simulink model "Relay_Blocks"  (Simulink 7.8)
settings: Solver=ode45  StartTime=0.0  StopTime=10.0  RelTol=1e-3
PreLoadFcn:
  | Ts = 1;
InitFcn:
  | Ts = 1;
undefined symbols (not defined in the file or in its folder): breakers_1ph_3ph, DiscIntNeverNeededParam, IEEE_Std_C37_112
libraries: simulink x12, powerlib_extras x8, lib_Timer_Counter x7, simulink_extras x3, dspsigops x1
settings Model: Creator=ma25949  LastModifiedBy=ma25949

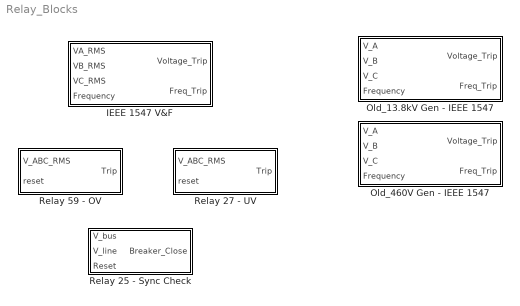
== system Relay_Blocks ==
  IEEE 1547 V&F : Subsystem  mask{V=13800, OF1=2, OF2=0.16, OV1=1, OV2=0.16, UF1=0.16, UF2=2, UV1=0.16, UV2=1, UV3=2}
      mask prompts: V "VoltageLL_RMS"; OF1 "OF1 (>60.5 Hz)"; OF2 "OF2 (>62 Hz)"; OV1 "OV1 (110% <V< 120% Vnom"; OV2 "OV2 (120% Vnom)"; UF1 "UF1 (<57 Hz)"; UF2 "UF2 (<59.5 Hz)"; UV1 "UV1 (<45% Vnom)"; UV2 "UV2 (45%<V<60% Vnom)"; UV3 "UV3 (60%<V<88% Vnom)"
      mask help:
      | This block implements interconnection system response according to IEEE Std. 1547-2014a.
      |
      | Fields to be filled are clearing times in seconds.
  Old_13.8kV Gen - IEEE 1547 : Subsystem  mask{OF1=2, OF2=0.16, OV1=1, OV2=0.16, UF1=0.16, UF2=2, UV1=0.16, UV2=1, UV3=2}
      mask prompts: OF1 "OF1 (>60.5 Hz)"; OF2 "OF2 (>62 Hz)"; OV1 "OV1 (110%<V<120% Vnom)"; OV2 "OV2 (>120% Vnom)"; UF1 "UF1 (<57 Hz)"; UF2 "UF2 (<59.5 Hz)"; UV1 "UV1 (<45% Vnom)"; UV2 "UV2 (45%<V<60% Vnom)"; UV3 "UV3 (60%<V<88% Vnom)"
      mask help:
      | This block implements interconnection system response according to IEEE Std. 1547-2014a.
      |
      | Fields to be filled are clearing times in seconds.
  Old_460V Gen - IEEE 1547 : Subsystem  mask{OF1=2, OF2=0.16, OV1=1, OV2=0.16, UF1=0.16, UF2=2, UV1=0.16, UV2=1, UV3=2}
      mask prompts: OF1 "OF1 (>60.5 Hz)"; OF2 "OF2 (>62 Hz)"; OV1 "OV1 (110%<V<120% Vnom)"; OV2 "OV2 (>120% Vnom)"; UF1 "UF1 (<57 Hz)"; UF2 "UF2 (<59.5 Hz)"; UV1 "UV1 (<45% Vnom)"; UV2 "UV2 (45%<V<60% Vnom)"; UV3 "UV3 (60%<V<88% Vnom)"
      mask help:
      | This block implements interconnection system response according to IEEE Std. 1547-2014a.
      |
      | Fields to be filled are clearing times in seconds.
  Relay 25 - Sync Check : Subsystem  mask{Cycles=2, V=13800}
      mask prompts: Cycles "# of cycles to check for sync"; V "VRMS_NominalV"
  Relay 27 - UV : Subsystem  mask{V=13800}
      mask prompts: V "Vnom"
      mask help: TOV Pickup is set to +15% of Vnominal.
  Relay 59 - OV : Subsystem  mask{V=13800}
      mask prompts: V "Vnom"
      mask help: TOV Pickup is set to +15% of Vnominal.

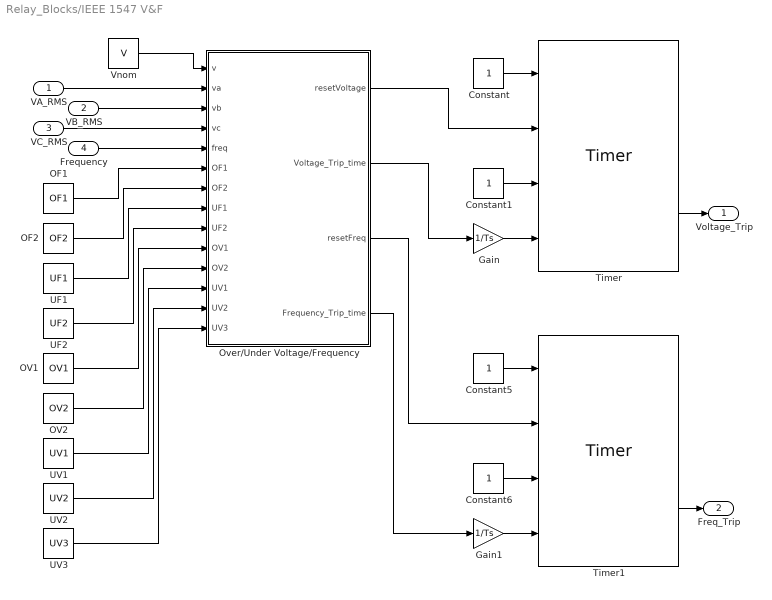
== system Relay_Blocks/IEEE 1547 V&F ==
  VA_RMS : Inport
  VB_RMS : Inport  Port=2
  VC_RMS : Inport  Port=3
  Frequency : Inport  Port=4
  Constant{,1,5..6} (4 alike) : Constant
  Gain : Gain  Gain=1/Ts
  Gain1 : Gain  Gain=1/Ts
  OF1 : Constant  Value=OF1
  OF2 : Constant  Value=OF2
  OV1 : Constant  Value=OV1
  OV2 : Constant  Value=OV2
  Over/Under Voltage/Frequency : MATLAB Function  TreatAsAtomicUnit=on
  Timer : lib_Timer_Counter/Timer
  Timer1 : lib_Timer_Counter/Timer
  UF1 : Constant  Value=UF1
  UF2 : Constant  Value=UF2
  UV1 : Constant  Value=UV1
  UV2 : Constant  Value=UV2
  UV3 : Constant  Value=UV3
  Vnom : Constant  Value=V
  Voltage_Trip : Outport
  Freq_Trip : Outport  Port=2
  wires:
  Constant/1 -> Timer/1
  Constant1/1 -> Timer/3
  Constant5/1 -> Timer1/1
  Constant6/1 -> Timer1/3
  Timer/2 -> Voltage_Trip/1
  Timer1/2 -> Freq_Trip/1
  VA_RMS/1 -> Over/Under Voltage/Frequency/2(va)
  Vnom/1 -> Over/Under Voltage/Frequency/1(v)
  VB_RMS/1 -> Over/Under Voltage/Frequency/3(vb)
  VC_RMS/1 -> Over/Under Voltage/Frequency/4(vc)
  Frequency/1 -> Over/Under Voltage/Frequency/5(freq)
  Over/Under Voltage/Frequency/1(resetVoltage) -> Timer/2
  Over/Under Voltage/Frequency/3(resetFreq) -> Timer1/2
  Gain1/1 -> Timer1/4
  Gain/1 -> Timer/4
  Over/Under Voltage/Frequency/2(Voltage_Trip_time) -> Gain/1
  Over/Under Voltage/Frequency/4(Frequency_Trip_time) -> Gain1/1
  OF1/1 -> Over/Under Voltage/Frequency/6(OF1)
  OF2/1 -> Over/Under Voltage/Frequency/7(OF2)
  UF1/1 -> Over/Under Voltage/Frequency/8(UF1)
  UF2/1 -> Over/Under Voltage/Frequency/9(UF2)
  OV1/1 -> Over/Under Voltage/Frequency/10(OV1)
  OV2/1 -> Over/Under Voltage/Frequency/11(OV2)
  UV1/1 -> Over/Under Voltage/Frequency/12(UV1)
  UV2/1 -> Over/Under Voltage/Frequency/13(UV2)
  UV3/1 -> Over/Under Voltage/Frequency/14(UV3)

== system Relay_Blocks/Old_13.8kV Gen - IEEE 1547 ==
  V_A : Inport
  V_B : Inport  Port=2
  V_C : Inport  Port=3
  Frequency : Inport  Port=4
  " Min_ClearingTime" : MinMax  Inputs=3
  Constant{,1,5..6} (4 alike) : Constant
  Frequency1 : Subsystem
  Logical Operator : Logic  Inputs=3  AllPortsSameDT=off  OutDataTypeStr=boolean
  PhaseA : Subsystem
  PhaseB : Subsystem
  PhaseC : Subsystem
  Timer : lib_Timer_Counter/Timer
  Timer1 : lib_Timer_Counter/Timer
  Voltage_Trip : Outport
  Freq_Trip : Outport  Port=2
  wires:
  Constant/1 -> Timer/1
  Constant1/1 -> Timer/3
  Constant5/1 -> Timer1/1
  Constant6/1 -> Timer1/3
  Frequency/1 -> Frequency1/1(Freq)
  Timer/2 -> Voltage_Trip/1
  Timer1/2 -> Freq_Trip/1
  V_A/1 -> PhaseA/1(V)
  V_B/1 -> PhaseB/1(V)
  V_C/1 -> PhaseC/1(V)
  PhaseA/2(Target Time) -> " Min_ClearingTime"/1
  " Min_ClearingTime"/1 -> Timer/4
  PhaseA/1(Reset) -> Logical Operator/1
  Logical Operator/1 -> Timer/2
  PhaseB/1(Reset) -> Logical Operator/2
  PhaseC/1(Reset) -> Logical Operator/3
  PhaseB/2(Target Time) -> " Min_ClearingTime"/2
  PhaseC/2(Target Time) -> " Min_ClearingTime"/3
  Frequency1/1(Reset) -> Timer1/2
  Frequency1/2(Target Time) -> Timer1/4

== system Relay_Blocks/Old_460V Gen - IEEE 1547 ==
  V_A : Inport
  V_B : Inport  Port=2
  V_C : Inport  Port=3
  Frequency : Inport  Port=4
  " Min_ClearingTime" : MinMax  Inputs=3
  Constant{,1,5..6} (4 alike) : Constant
  Frequency1 : Subsystem
  Logical Operator : Logic  Inputs=3  AllPortsSameDT=off  OutDataTypeStr=boolean
  PhaseA : Subsystem
  PhaseB : Subsystem
  PhaseC : Subsystem
  Timer : lib_Timer_Counter/Timer
  Timer1 : lib_Timer_Counter/Timer
  Voltage_Trip : Outport
  Freq_Trip : Outport  Port=2
  wires:
  Constant/1 -> Timer/1
  Constant1/1 -> Timer/3
  Constant5/1 -> Timer1/1
  Constant6/1 -> Timer1/3
  Frequency/1 -> Frequency1/1(Freq)
  Timer/2 -> Voltage_Trip/1
  Timer1/2 -> Freq_Trip/1
  V_A/1 -> PhaseA/1(V)
  V_B/1 -> PhaseB/1(V)
  V_C/1 -> PhaseC/1(V)
  PhaseA/2(Target Time) -> " Min_ClearingTime"/1
  " Min_ClearingTime"/1 -> Timer/4
  PhaseA/1(Reset) -> Logical Operator/1
  Logical Operator/1 -> Timer/2
  PhaseB/1(Reset) -> Logical Operator/2
  PhaseC/1(Reset) -> Logical Operator/3
  PhaseB/2(Target Time) -> " Min_ClearingTime"/2
  PhaseC/2(Target Time) -> " Min_ClearingTime"/3
  Frequency1/1(Reset) -> Timer1/2
  Frequency1/2(Target Time) -> Timer1/4

== system Relay_Blocks/Relay 25 - Sync Check ==
  V_bus : Inport
  V_line : Inport  Port=2
  Reset : Inport  Port=3
  Compare To Constant3 : simulink/Logic and Bit Operations/Compare To Constant  relop===  const=0  OutDataTypeStr=uint8
  Constant : Constant
  Freq_Comparator : Subsystem
  Gain : Gain  Gain=0.16667/Ts
  Logical Operator : Logic  Inputs=3  AllPortsSameDT=off  OutDataTypeStr=boolean
  Logical Operator1 : Logic  Operator=OR  AllPortsSameDT=off  OutDataTypeStr=boolean
  Phase_Comparator : Subsystem
  RMS Calculator1 : Subsystem
  RMS Calculator2 : Subsystem
  Subsystem : Subsystem
  Target_time : Constant  Value=Cycles
  Timer : lib_Timer_Counter/Timer
  Voltage_Comparator : Subsystem
  Breaker_Close : Outport
  wires:
  Logical Operator/1 -> Compare To Constant3/1, Timer/1
  Constant/1 -> Timer/3
  Phase_Comparator/2(Locked) -> Logical Operator/3
  Freq_Comparator/2(Locked) -> Logical Operator/2
  Voltage_Comparator/3(Locked) -> Logical Operator/1
  RMS Calculator1/1(VRMSLL) -> Voltage_Comparator/2(V_line)
  Subsystem/4(wt_line) -> Phase_Comparator/2(wt_line)
  Subsystem/3(wt_bus) -> Phase_Comparator/1(wt_bus)
  Subsystem/2(f_line) -> Freq_Comparator/2(f_line)
  Subsystem/1(f_bus) -> Freq_Comparator/1(f_bus)
  V_line/1 -> Subsystem/2(V_line), RMS Calculator1/1(Vpeak)
  V_bus/1 -> Subsystem/1(V_bus), RMS Calculator2/1(Vpeak)
  Timer/2 -> Breaker_Close/1
  RMS Calculator2/1(VRMSLL) -> Voltage_Comparator/1(V_bus)
  ? -> [Mode]
  Target_time/1 -> Gain/1
  Gain/1 -> Timer/4
  Reset/1 -> Logical Operator1/1
  Logical Operator1/1 -> Timer/2
  Compare To Constant3/1 -> Logical Operator1/2

== system Relay_Blocks/Relay 27 - UV ==
  V_ABC_RMS : Inport
  reset : Inport  Port=2
  Data Type Conversion1 : DataTypeConversion
  Data Type Conversion3 : DataTypeConversion
  Demux : Demux  Outputs=3
  Demux1 : Demux  Outputs=3
  Discrete-Time Integrator1 : DiscreteIntegrator  IntegratorMethod=Integration: Trapezoidal  ExternalReset=falling  InitialConditionMode=State only (most efficient)  SampleTime=-1  ICPrevOutput=DiscIntNeverNeededParam  ICPrevScaledInput=DiscIntNeverNeededParam
  Gain : Gain  Gain=0.85
  Logical Operator1 : Logic  Operator=OR  Inputs=3  AllPortsSameDT=off  OutDataTypeStr=boolean
  Relational Operator : RelationalOperator  Operator=<  OutDataTypeStr=boolean
  Relational Operator1 : RelationalOperator  Operator=>  OutDataTypeStr=boolean
  S-R Flip-Flop : simulink_extras/Flip Flops/S-R Flip-Flop  initial_condition=0
  Terminator : Terminator
  UV Relay : Subsystem  AncestorBlock=breakers_1ph_3ph/IEEE_Std_C37_112
  Vnom : Constant  Value=V
  Trip : Outport
  wires:
  Data Type Conversion1/1 -> Discrete-Time Integrator1/1
  UV Relay/1(T_trip) -> Relational Operator/1  "t_trip"
  Demux/1 -> UV Relay/2(Va)
  Demux/2 -> UV Relay/3(Vb)
  Demux/3 -> UV Relay/4(Vc)
  V_ABC_RMS/1 -> Demux/1, Relational Operator1/2
  S-R Flip-Flop/1 -> Trip/1
  S-R Flip-Flop/2 -> Terminator/1
  reset/1 -> Data Type Conversion3/1
  Data Type Conversion3/1 -> S-R Flip-Flop/2
  Relational Operator1/1 -> Data Type Conversion1/1, Discrete-Time Integrator1/2
  Discrete-Time Integrator1/1 -> Relational Operator/2
  Vnom/1 -> Gain/1
  Gain/1 -> UV Relay/1(TOV_pickup), Relational Operator1/1
  Relational Operator/1 -> Demux1/1
  Demux1/1 -> Logical Operator1/1
  Demux1/2 -> Logical Operator1/2
  Demux1/3 -> Logical Operator1/3
  Logical Operator1/1 -> S-R Flip-Flop/1

== system Relay_Blocks/Relay 59 - OV ==
  V_ABC_RMS : Inport
  reset : Inport  Port=2
  Data Type Conversion1 : DataTypeConversion
  Data Type Conversion3 : DataTypeConversion
  Demux : Demux  Outputs=3
  Demux1 : Demux  Outputs=3
  Discrete-Time Integrator1 : DiscreteIntegrator  IntegratorMethod=Integration: Trapezoidal  ExternalReset=falling  InitialConditionMode=State only (most efficient)  SampleTime=-1  ICPrevOutput=DiscIntNeverNeededParam  ICPrevScaledInput=DiscIntNeverNeededParam
  Gain : Gain  Gain=1.15
  Logical Operator1 : Logic  Operator=OR  Inputs=3  AllPortsSameDT=off  OutDataTypeStr=boolean
  OV Relay : Subsystem  AncestorBlock=breakers_1ph_3ph/IEEE_Std_C37_112
  Relational Operator : RelationalOperator  Operator=<  OutDataTypeStr=boolean
  Relational Operator1 : RelationalOperator  Operator=<  OutDataTypeStr=boolean
  S-R Flip-Flop : simulink_extras/Flip Flops/S-R Flip-Flop  initial_condition=0
  Terminator : Terminator
  Vnom : Constant  Value=V
  Trip : Outport
  wires:
  Data Type Conversion1/1 -> Discrete-Time Integrator1/1
  OV Relay/1(T_trip) -> Relational Operator/1  "t_trip"
  Demux/1 -> OV Relay/2(Va)
  Demux/2 -> OV Relay/3(Vb)
  Demux/3 -> OV Relay/4(Vc)
  V_ABC_RMS/1 -> Demux/1, Relational Operator1/2
  S-R Flip-Flop/1 -> Trip/1
  S-R Flip-Flop/2 -> Terminator/1
  reset/1 -> Data Type Conversion3/1
  Data Type Conversion3/1 -> S-R Flip-Flop/2
  Relational Operator1/1 -> Data Type Conversion1/1, Discrete-Time Integrator1/2
  Discrete-Time Integrator1/1 -> Relational Operator/2
  Vnom/1 -> Gain/1
  Gain/1 -> OV Relay/1(TOV_pickup), Relational Operator1/1
  Relational Operator/1 -> Demux1/1
  Demux1/1 -> Logical Operator1/1
  Demux1/2 -> Logical Operator1/2
  Demux1/3 -> Logical Operator1/3
  Logical Operator1/1 -> S-R Flip-Flop/1

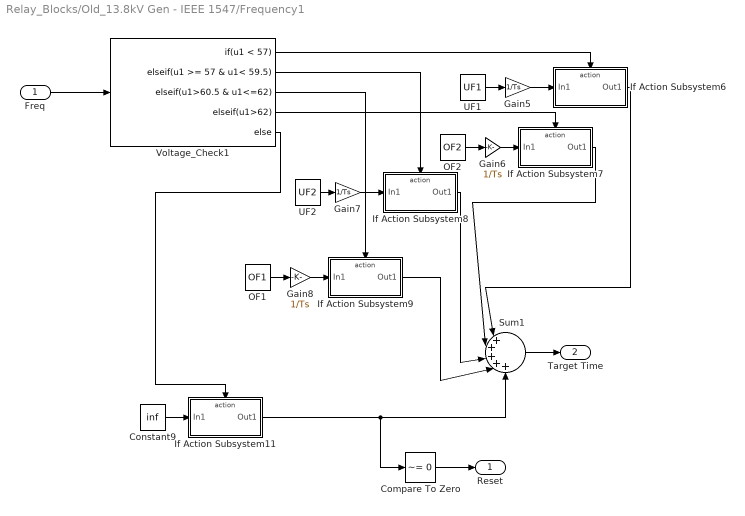
== system Relay_Blocks/Old_13.8kV Gen - IEEE 1547/Frequency1 ==
  Freq : Inport
  Compare To Zero : simulink/Logic and Bit Operations/Compare To Zero  relop=~=  OutDataTypeStr=uint8
  Constant9 : Constant  Value=inf
  Gain{5..8} (4 alike) : Gain  Gain=1/Ts
  If Action Subsystem11 : Subsystem  TreatAsAtomicUnit=on
  If Action Subsystem6 : Subsystem  TreatAsAtomicUnit=on
  If Action Subsystem7 : Subsystem  TreatAsAtomicUnit=on
  If Action Subsystem8 : Subsystem  TreatAsAtomicUnit=on
  If Action Subsystem9 : Subsystem  TreatAsAtomicUnit=on
  OF1 : Constant  Value=OF1
  OF2 : Constant  Value=OF2
  Sum1 : Sum  Inputs=|+++++
  UF1 : Constant  Value=UF1
  UF2 : Constant  Value=UF2
  Voltage_Check1 : If  IfExpression=u1 < 57  ElseIfExpressions="u1 >= 57 & u1< 59.5,  u1>60.5 & u1<=62, u1>62"
  Reset : Outport
  Target Time : Outport  Port=2
  wires:
  Freq/1 -> Voltage_Check1/1
  Voltage_Check1/1 -> If Action Subsystem6/Action
  UF1/1 -> Gain5/1
  Voltage_Check1/4 -> If Action Subsystem7/Action
  Voltage_Check1/2 -> If Action Subsystem8/Action
  Voltage_Check1/3 -> If Action Subsystem9/Action
  UF2/1 -> Gain7/1
  Voltage_Check1/5 -> If Action Subsystem11/Action
  Constant9/1 -> If Action Subsystem11/1(In1)
  If Action Subsystem6/1(Out1) -> Sum1/1
  If Action Subsystem7/1(Out1) -> Sum1/2
  If Action Subsystem8/1(Out1) -> Sum1/3
  If Action Subsystem9/1(Out1) -> Sum1/4
  If Action Subsystem11/1(Out1) -> Sum1/5, Compare To Zero/1
  OF1/1 -> Gain8/1
  OF2/1 -> Gain6/1
  Gain5/1 -> If Action Subsystem6/1(In1)
  Gain6/1 -> If Action Subsystem7/1(In1)
  Gain7/1 -> If Action Subsystem8/1(In1)
  Gain8/1 -> If Action Subsystem9/1(In1)
  Sum1/1 -> Target Time/1
  Compare To Zero/1 -> Reset/1

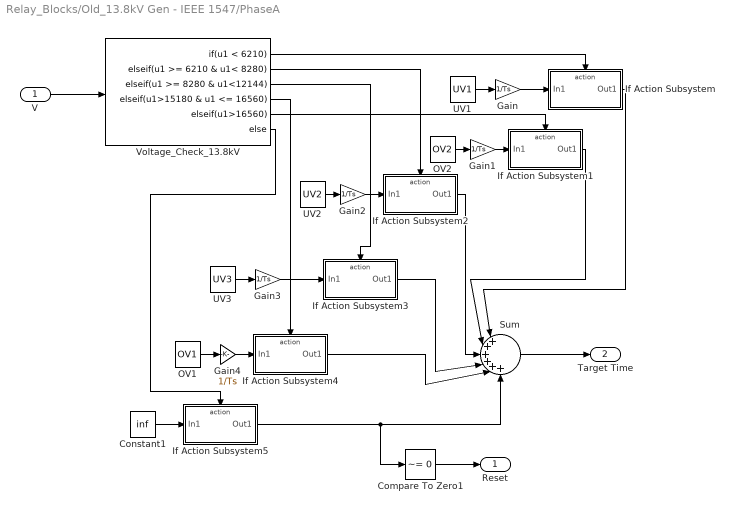
== system Relay_Blocks/Old_13.8kV Gen - IEEE 1547/PhaseA ==
  V : Inport
  Compare To Zero1 : simulink/Logic and Bit Operations/Compare To Zero  relop=~=  OutDataTypeStr=uint8
  Constant1 : Constant  Value=inf
  Gain{,1..4} (5 alike) : Gain  Gain=1/Ts
  If Action Subsystem : Subsystem  TreatAsAtomicUnit=on
  If Action Subsystem1 : Subsystem  TreatAsAtomicUnit=on
  If Action Subsystem2 : Subsystem  TreatAsAtomicUnit=on
  If Action Subsystem3 : Subsystem  TreatAsAtomicUnit=on
  If Action Subsystem4 : Subsystem  TreatAsAtomicUnit=on
  If Action Subsystem5 : Subsystem  TreatAsAtomicUnit=on
  OV1 : Constant  Value=OV1
  OV2 : Constant  Value=OV2
  Sum : Sum  Inputs=|++++++
  UV1 : Constant  Value=UV1
  UV2 : Constant  Value=UV2
  UV3 : Constant  Value=UV3
  Voltage_Check_13.8kV : If  IfExpression=u1 < 6210  ElseIfExpressions="u1 >= 6210 & u1< 8280,  u1 >= 8280 & u1<12144, u1>15180 & u1 <= 16560, u1>16560"
  Reset : Outport
  Target Time : Outport  Port=2
  wires:
  Voltage_Check_13.8kV/1 -> If Action Subsystem/Action
  Voltage_Check_13.8kV/5 -> If Action Subsystem1/Action
  Voltage_Check_13.8kV/2 -> If Action Subsystem2/Action
  Voltage_Check_13.8kV/3 -> If Action Subsystem3/Action
  Voltage_Check_13.8kV/4 -> If Action Subsystem4/Action
  UV3/1 -> Gain3/1
  Voltage_Check_13.8kV/6 -> If Action Subsystem5/Action
  Constant1/1 -> If Action Subsystem5/1(In1)
  If Action Subsystem/1(Out1) -> Sum/1
  If Action Subsystem1/1(Out1) -> Sum/2
  If Action Subsystem2/1(Out1) -> Sum/3
  If Action Subsystem3/1(Out1) -> Sum/4
  If Action Subsystem4/1(Out1) -> Sum/5
  If Action Subsystem5/1(Out1) -> Sum/6, Compare To Zero1/1
  OV1/1 -> Gain4/1
  UV1/1 -> Gain/1
  Gain/1 -> If Action Subsystem/1(In1)
  OV2/1 -> Gain1/1
  Gain1/1 -> If Action Subsystem1/1(In1)
  UV2/1 -> Gain2/1
  Gain2/1 -> If Action Subsystem2/1(In1)
  Gain3/1 -> If Action Subsystem3/1(In1)
  Gain4/1 -> If Action Subsystem4/1(In1)
  V/1 -> Voltage_Check_13.8kV/1
  Compare To Zero1/1 -> Reset/1
  Sum/1 -> Target Time/1

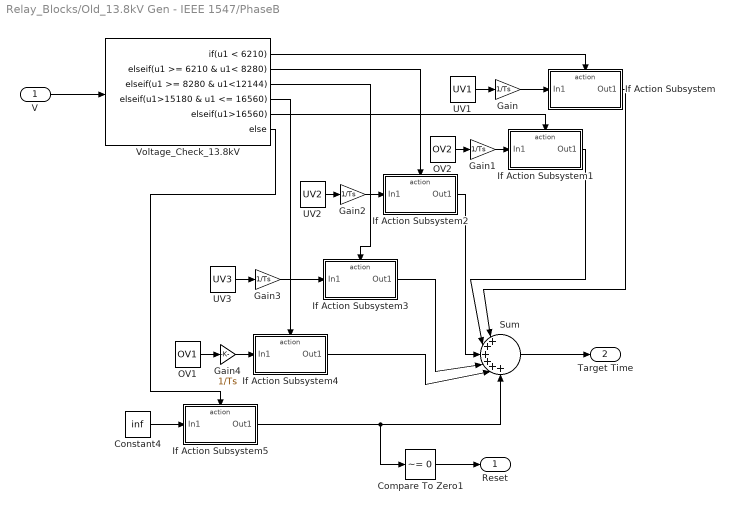
== system Relay_Blocks/Old_13.8kV Gen - IEEE 1547/PhaseB ==
  V : Inport
  Compare To Zero1 : simulink/Logic and Bit Operations/Compare To Zero  relop=~=  OutDataTypeStr=uint8
  Constant4 : Constant  Value=inf
  Gain{,1..4} (5 alike) : Gain  Gain=1/Ts
  If Action Subsystem : Subsystem  TreatAsAtomicUnit=on
  If Action Subsystem1 : Subsystem  TreatAsAtomicUnit=on
  If Action Subsystem2 : Subsystem  TreatAsAtomicUnit=on
  If Action Subsystem3 : Subsystem  TreatAsAtomicUnit=on
  If Action Subsystem4 : Subsystem  TreatAsAtomicUnit=on
  If Action Subsystem5 : Subsystem  TreatAsAtomicUnit=on
  OV1 : Constant  Value=OV1
  OV2 : Constant  Value=OV2
  Sum : Sum  Inputs=|++++++
  UV1 : Constant  Value=UV1
  UV2 : Constant  Value=UV2
  UV3 : Constant  Value=UV3
  Voltage_Check_13.8kV : If  IfExpression=u1 < 6210  ElseIfExpressions="u1 >= 6210 & u1< 8280,  u1 >= 8280 & u1<12144, u1>15180 & u1 <= 16560, u1>16560"
  Reset : Outport
  Target Time : Outport  Port=2
  wires:
  Voltage_Check_13.8kV/1 -> If Action Subsystem/Action
  Voltage_Check_13.8kV/5 -> If Action Subsystem1/Action
  Voltage_Check_13.8kV/2 -> If Action Subsystem2/Action
  Voltage_Check_13.8kV/3 -> If Action Subsystem3/Action
  Voltage_Check_13.8kV/4 -> If Action Subsystem4/Action
  UV3/1 -> Gain3/1
  Voltage_Check_13.8kV/6 -> If Action Subsystem5/Action
  Constant4/1 -> If Action Subsystem5/1(In1)
  If Action Subsystem/1(Out1) -> Sum/1
  If Action Subsystem1/1(Out1) -> Sum/2
  If Action Subsystem2/1(Out1) -> Sum/3
  If Action Subsystem4/1(Out1) -> Sum/5
  If Action Subsystem5/1(Out1) -> Sum/6, Compare To Zero1/1
  OV1/1 -> Gain4/1
  UV1/1 -> Gain/1
  Gain/1 -> If Action Subsystem/1(In1)
  OV2/1 -> Gain1/1
  Gain1/1 -> If Action Subsystem1/1(In1)
  UV2/1 -> Gain2/1
  Gain2/1 -> If Action Subsystem2/1(In1)
  Gain3/1 -> If Action Subsystem3/1(In1)
  Gain4/1 -> If Action Subsystem4/1(In1)
  V/1 -> Voltage_Check_13.8kV/1
  Compare To Zero1/1 -> Reset/1
  Sum/1 -> Target Time/1
  If Action Subsystem3/1(Out1) -> Sum/4

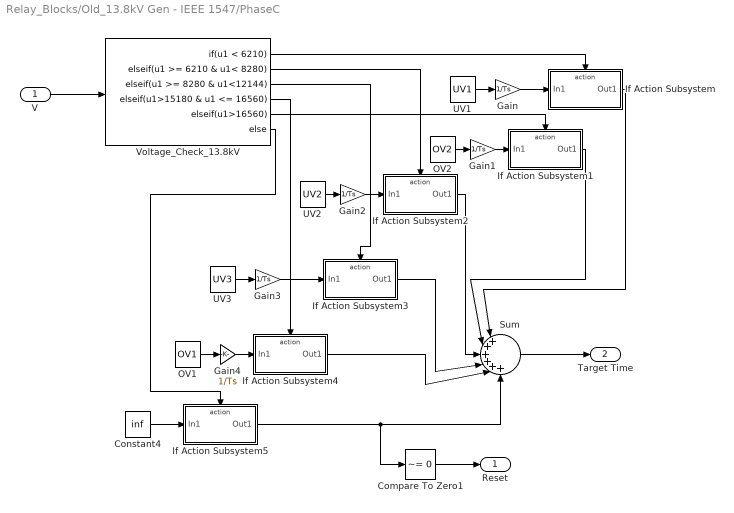
== system Relay_Blocks/Old_13.8kV Gen - IEEE 1547/PhaseC ==
  V : Inport
  Compare To Zero1 : simulink/Logic and Bit Operations/Compare To Zero  relop=~=  OutDataTypeStr=uint8
  Constant4 : Constant  Value=inf
  Gain{,1..4} (5 alike) : Gain  Gain=1/Ts
  If Action Subsystem : Subsystem  TreatAsAtomicUnit=on
  If Action Subsystem1 : Subsystem  TreatAsAtomicUnit=on
  If Action Subsystem2 : Subsystem  TreatAsAtomicUnit=on
  If Action Subsystem3 : Subsystem  TreatAsAtomicUnit=on
  If Action Subsystem4 : Subsystem  TreatAsAtomicUnit=on
  If Action Subsystem5 : Subsystem  TreatAsAtomicUnit=on
  OV1 : Constant  Value=OV1
  OV2 : Constant  Value=OV2
  Sum : Sum  Inputs=|++++++
  UV1 : Constant  Value=UV1
  UV2 : Constant  Value=UV2
  UV3 : Constant  Value=UV3
  Voltage_Check_13.8kV : If  IfExpression=u1 < 6210  ElseIfExpressions="u1 >= 6210 & u1< 8280,  u1 >= 8280 & u1<12144, u1>15180 & u1 <= 16560, u1>16560"
  Reset : Outport
  Target Time : Outport  Port=2
  wires:
  Voltage_Check_13.8kV/1 -> If Action Subsystem/Action
  Voltage_Check_13.8kV/5 -> If Action Subsystem1/Action
  Voltage_Check_13.8kV/2 -> If Action Subsystem2/Action
  Voltage_Check_13.8kV/3 -> If Action Subsystem3/Action
  Voltage_Check_13.8kV/4 -> If Action Subsystem4/Action
  UV3/1 -> Gain3/1
  Voltage_Check_13.8kV/6 -> If Action Subsystem5/Action
  Constant4/1 -> If Action Subsystem5/1(In1)
  If Action Subsystem/1(Out1) -> Sum/1
  If Action Subsystem1/1(Out1) -> Sum/2
  If Action Subsystem2/1(Out1) -> Sum/3
  If Action Subsystem3/1(Out1) -> Sum/4
  If Action Subsystem4/1(Out1) -> Sum/5
  If Action Subsystem5/1(Out1) -> Sum/6, Compare To Zero1/1
  OV1/1 -> Gain4/1
  UV1/1 -> Gain/1
  Gain/1 -> If Action Subsystem/1(In1)
  OV2/1 -> Gain1/1
  Gain1/1 -> If Action Subsystem1/1(In1)
  UV2/1 -> Gain2/1
  Gain2/1 -> If Action Subsystem2/1(In1)
  Gain3/1 -> If Action Subsystem3/1(In1)
  Gain4/1 -> If Action Subsystem4/1(In1)
  V/1 -> Voltage_Check_13.8kV/1
  Compare To Zero1/1 -> Reset/1
  Sum/1 -> Target Time/1

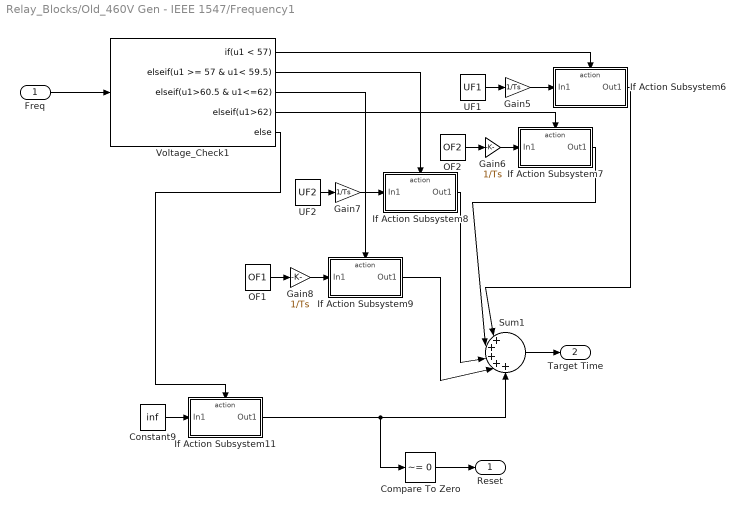
== system Relay_Blocks/Old_460V Gen - IEEE 1547/Frequency1 ==
  Freq : Inport
  Compare To Zero : simulink/Logic and Bit Operations/Compare To Zero  relop=~=  OutDataTypeStr=uint8
  Constant9 : Constant  Value=inf
  Gain{5..8} (4 alike) : Gain  Gain=1/Ts
  If Action Subsystem11 : Subsystem  TreatAsAtomicUnit=on
  If Action Subsystem6 : Subsystem  TreatAsAtomicUnit=on
  If Action Subsystem7 : Subsystem  TreatAsAtomicUnit=on
  If Action Subsystem8 : Subsystem  TreatAsAtomicUnit=on
  If Action Subsystem9 : Subsystem  TreatAsAtomicUnit=on
  OF1 : Constant  Value=OF1
  OF2 : Constant  Value=OF2
  Sum1 : Sum  Inputs=|+++++
  UF1 : Constant  Value=UF1
  UF2 : Constant  Value=UF2
  Voltage_Check1 : If  IfExpression=u1 < 57  ElseIfExpressions="u1 >= 57 & u1< 59.5,  u1>60.5 & u1<=62, u1>62"
  Reset : Outport
  Target Time : Outport  Port=2
  wires:
  Freq/1 -> Voltage_Check1/1
  Voltage_Check1/1 -> If Action Subsystem6/Action
  UF1/1 -> Gain5/1
  Voltage_Check1/4 -> If Action Subsystem7/Action
  Voltage_Check1/2 -> If Action Subsystem8/Action
  Voltage_Check1/3 -> If Action Subsystem9/Action
  UF2/1 -> Gain7/1
  Voltage_Check1/5 -> If Action Subsystem11/Action
  Constant9/1 -> If Action Subsystem11/1(In1)
  If Action Subsystem6/1(Out1) -> Sum1/1
  If Action Subsystem7/1(Out1) -> Sum1/2
  If Action Subsystem8/1(Out1) -> Sum1/3
  If Action Subsystem9/1(Out1) -> Sum1/4
  If Action Subsystem11/1(Out1) -> Sum1/5, Compare To Zero/1
  OF1/1 -> Gain8/1
  OF2/1 -> Gain6/1
  Gain5/1 -> If Action Subsystem6/1(In1)
  Gain6/1 -> If Action Subsystem7/1(In1)
  Gain7/1 -> If Action Subsystem8/1(In1)
  Gain8/1 -> If Action Subsystem9/1(In1)
  Sum1/1 -> Target Time/1
  Compare To Zero/1 -> Reset/1

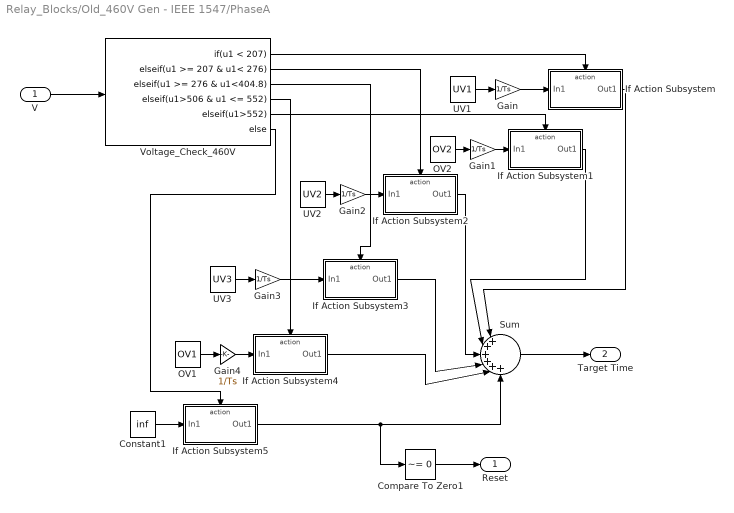
== system Relay_Blocks/Old_460V Gen - IEEE 1547/PhaseA ==
  V : Inport
  Compare To Zero1 : simulink/Logic and Bit Operations/Compare To Zero  relop=~=  OutDataTypeStr=uint8
  Constant1 : Constant  Value=inf
  Gain{,1..4} (5 alike) : Gain  Gain=1/Ts
  If Action Subsystem : Subsystem  TreatAsAtomicUnit=on
  If Action Subsystem1 : Subsystem  TreatAsAtomicUnit=on
  If Action Subsystem2 : Subsystem  TreatAsAtomicUnit=on
  If Action Subsystem3 : Subsystem  TreatAsAtomicUnit=on
  If Action Subsystem4 : Subsystem  TreatAsAtomicUnit=on
  If Action Subsystem5 : Subsystem  TreatAsAtomicUnit=on
  OV1 : Constant  Value=OV1
  OV2 : Constant  Value=OV2
  Sum : Sum  Inputs=|++++++
  UV1 : Constant  Value=UV1
  UV2 : Constant  Value=UV2
  UV3 : Constant  Value=UV3
  Voltage_Check_460V : If  IfExpression=u1 < 207  ElseIfExpressions="u1 >= 207 & u1< 276,  u1 >= 276 & u1<404.8, u1>506 & u1 <= 552, u1>552"
  Reset : Outport
  Target Time : Outport  Port=2
  wires:
  Voltage_Check_460V/1 -> If Action Subsystem/Action
  Voltage_Check_460V/5 -> If Action Subsystem1/Action
  Voltage_Check_460V/2 -> If Action Subsystem2/Action
  Voltage_Check_460V/3 -> If Action Subsystem3/Action
  Voltage_Check_460V/4 -> If Action Subsystem4/Action
  UV3/1 -> Gain3/1
  Voltage_Check_460V/6 -> If Action Subsystem5/Action
  Constant1/1 -> If Action Subsystem5/1(In1)
  If Action Subsystem/1(Out1) -> Sum/1
  If Action Subsystem1/1(Out1) -> Sum/2
  If Action Subsystem2/1(Out1) -> Sum/3
  If Action Subsystem3/1(Out1) -> Sum/4
  If Action Subsystem4/1(Out1) -> Sum/5
  If Action Subsystem5/1(Out1) -> Sum/6, Compare To Zero1/1
  OV1/1 -> Gain4/1
  UV1/1 -> Gain/1
  Gain/1 -> If Action Subsystem/1(In1)
  OV2/1 -> Gain1/1
  Gain1/1 -> If Action Subsystem1/1(In1)
  UV2/1 -> Gain2/1
  Gain2/1 -> If Action Subsystem2/1(In1)
  Gain3/1 -> If Action Subsystem3/1(In1)
  Gain4/1 -> If Action Subsystem4/1(In1)
  V/1 -> Voltage_Check_460V/1
  Compare To Zero1/1 -> Reset/1
  Sum/1 -> Target Time/1

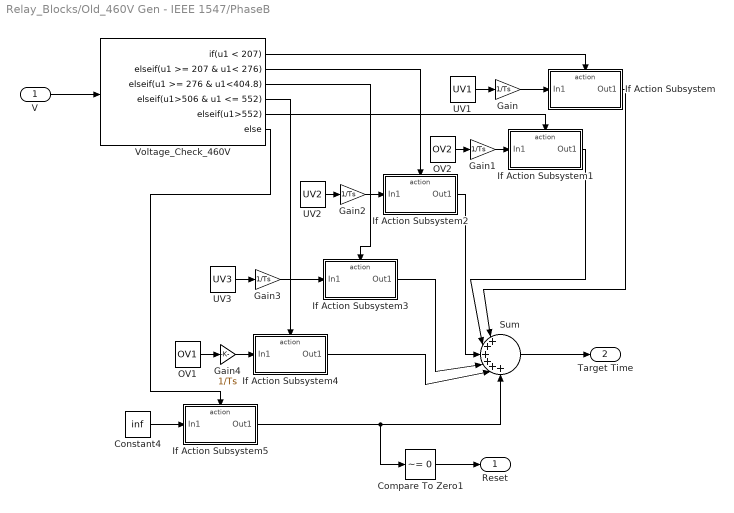
== system Relay_Blocks/Old_460V Gen - IEEE 1547/PhaseB ==
  V : Inport
  Compare To Zero1 : simulink/Logic and Bit Operations/Compare To Zero  relop=~=  OutDataTypeStr=uint8
  Constant4 : Constant  Value=inf
  Gain{,1..4} (5 alike) : Gain  Gain=1/Ts
  If Action Subsystem : Subsystem  TreatAsAtomicUnit=on
  If Action Subsystem1 : Subsystem  TreatAsAtomicUnit=on
  If Action Subsystem2 : Subsystem  TreatAsAtomicUnit=on
  If Action Subsystem3 : Subsystem  TreatAsAtomicUnit=on
  If Action Subsystem4 : Subsystem  TreatAsAtomicUnit=on
  If Action Subsystem5 : Subsystem  TreatAsAtomicUnit=on
  OV1 : Constant  Value=OV1
  OV2 : Constant  Value=OV2
  Sum : Sum  Inputs=|++++++
  UV1 : Constant  Value=UV1
  UV2 : Constant  Value=UV2
  UV3 : Constant  Value=UV3
  Voltage_Check_460V : If  IfExpression=u1 < 207  ElseIfExpressions="u1 >= 207 & u1< 276,  u1 >= 276 & u1<404.8, u1>506 & u1 <= 552, u1>552"
  Reset : Outport
  Target Time : Outport  Port=2
  wires:
  Voltage_Check_460V/1 -> If Action Subsystem/Action
  Voltage_Check_460V/5 -> If Action Subsystem1/Action
  Voltage_Check_460V/2 -> If Action Subsystem2/Action
  Voltage_Check_460V/3 -> If Action Subsystem3/Action
  Voltage_Check_460V/4 -> If Action Subsystem4/Action
  UV3/1 -> Gain3/1
  Voltage_Check_460V/6 -> If Action Subsystem5/Action
  Constant4/1 -> If Action Subsystem5/1(In1)
  If Action Subsystem/1(Out1) -> Sum/1
  If Action Subsystem1/1(Out1) -> Sum/2
  If Action Subsystem2/1(Out1) -> Sum/3
  If Action Subsystem4/1(Out1) -> Sum/5
  If Action Subsystem5/1(Out1) -> Sum/6, Compare To Zero1/1
  OV1/1 -> Gain4/1
  UV1/1 -> Gain/1
  Gain/1 -> If Action Subsystem/1(In1)
  OV2/1 -> Gain1/1
  Gain1/1 -> If Action Subsystem1/1(In1)
  UV2/1 -> Gain2/1
  Gain2/1 -> If Action Subsystem2/1(In1)
  Gain3/1 -> If Action Subsystem3/1(In1)
  Gain4/1 -> If Action Subsystem4/1(In1)
  V/1 -> Voltage_Check_460V/1
  Compare To Zero1/1 -> Reset/1
  Sum/1 -> Target Time/1
  If Action Subsystem3/1(Out1) -> Sum/4

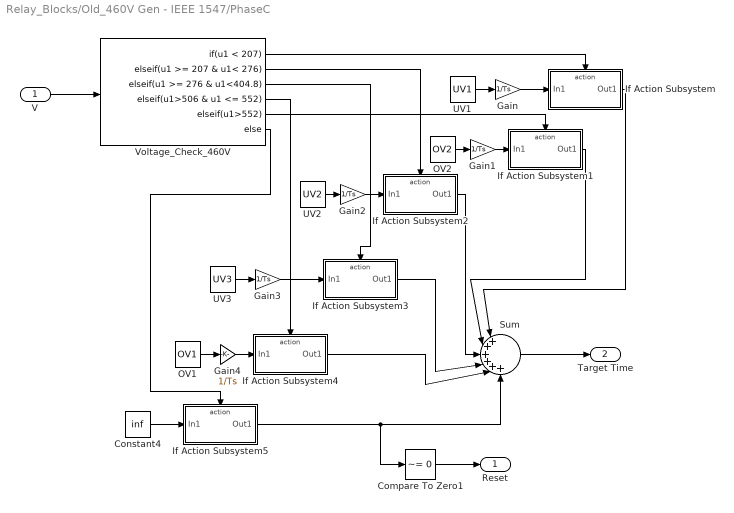
== system Relay_Blocks/Old_460V Gen - IEEE 1547/PhaseC ==
  V : Inport
  Compare To Zero1 : simulink/Logic and Bit Operations/Compare To Zero  relop=~=  OutDataTypeStr=uint8
  Constant4 : Constant  Value=inf
  Gain{,1..4} (5 alike) : Gain  Gain=1/Ts
  If Action Subsystem : Subsystem  TreatAsAtomicUnit=on
  If Action Subsystem1 : Subsystem  TreatAsAtomicUnit=on
  If Action Subsystem2 : Subsystem  TreatAsAtomicUnit=on
  If Action Subsystem3 : Subsystem  TreatAsAtomicUnit=on
  If Action Subsystem4 : Subsystem  TreatAsAtomicUnit=on
  If Action Subsystem5 : Subsystem  TreatAsAtomicUnit=on
  OV1 : Constant  Value=OV1
  OV2 : Constant  Value=OV2
  Sum : Sum  Inputs=|++++++
  UV1 : Constant  Value=UV1
  UV2 : Constant  Value=UV2
  UV3 : Constant  Value=UV3
  Voltage_Check_460V : If  IfExpression=u1 < 207  ElseIfExpressions="u1 >= 207 & u1< 276,  u1 >= 276 & u1<404.8, u1>506 & u1 <= 552, u1>552"
  Reset : Outport
  Target Time : Outport  Port=2
  wires:
  Voltage_Check_460V/1 -> If Action Subsystem/Action
  Voltage_Check_460V/5 -> If Action Subsystem1/Action
  Voltage_Check_460V/2 -> If Action Subsystem2/Action
  Voltage_Check_460V/3 -> If Action Subsystem3/Action
  Voltage_Check_460V/4 -> If Action Subsystem4/Action
  UV3/1 -> Gain3/1
  Voltage_Check_460V/6 -> If Action Subsystem5/Action
  Constant4/1 -> If Action Subsystem5/1(In1)
  If Action Subsystem/1(Out1) -> Sum/1
  If Action Subsystem1/1(Out1) -> Sum/2
  If Action Subsystem2/1(Out1) -> Sum/3
  If Action Subsystem3/1(Out1) -> Sum/4
  If Action Subsystem4/1(Out1) -> Sum/5
  If Action Subsystem5/1(Out1) -> Sum/6, Compare To Zero1/1
  OV1/1 -> Gain4/1
  UV1/1 -> Gain/1
  Gain/1 -> If Action Subsystem/1(In1)
  OV2/1 -> Gain1/1
  Gain1/1 -> If Action Subsystem1/1(In1)
  UV2/1 -> Gain2/1
  Gain2/1 -> If Action Subsystem2/1(In1)
  Gain3/1 -> If Action Subsystem3/1(In1)
  Gain4/1 -> If Action Subsystem4/1(In1)
  V/1 -> Voltage_Check_460V/1
  Compare To Zero1/1 -> Reset/1
  Sum/1 -> Target Time/1

== system Relay_Blocks/Relay 25 - Sync Check/Freq_Comparator ==
  f_bus : Inport
  f_line : Inport  Port=2
  Abs : Abs
  Compare To Constant2 : simulink/Logic and Bit Operations/Compare To Constant  relop=<=  const=0.2  OutDataTypeStr=uint8
  Demux : Demux  Outputs=3
  Demux1 : Demux  Outputs=3
  Demux2 : Demux  Outputs=3
  Fcn1 : Fcn  Expr=u(2)-u(1)
  Fcn2 : Fcn  Expr=u(2)-u(1)
  Fcn3 : Fcn  Expr=u(2)-u(1)
  Logical Operator : Logic  Inputs=3  AllPortsSameDT=off  OutDataTypeStr=boolean
  Mux : Mux  Inputs=2
  Mux1 : Mux  Inputs=2
  Mux2 : Mux  Inputs=2
  Mux3 : Mux  Inputs=3
  Diff : Outport
  Locked : Outport  Port=2
  wires:
  Abs/1 -> Compare To Constant2/1
  f_line/1 -> Demux1/1
  f_bus/1 -> Demux/1
  Demux/1 -> Mux/1
  Demux1/1 -> Mux/2
  Mux/1 -> Fcn2/1
  Demux/2 -> Mux1/1
  Demux1/2 -> Mux1/2
  Demux/3 -> Mux2/1
  Demux1/3 -> Mux2/2
  Mux1/1 -> Fcn1/1
  Mux2/1 -> Fcn3/1
  Fcn2/1 -> Mux3/1
  Fcn1/1 -> Mux3/2
  Fcn3/1 -> Mux3/3
  Mux3/1 -> Abs/1, Diff/1
  Compare To Constant2/1 -> Demux2/1
  Demux2/1 -> Logical Operator/1
  Demux2/2 -> Logical Operator/2
  Demux2/3 -> Logical Operator/3
  Logical Operator/1 -> Locked/1

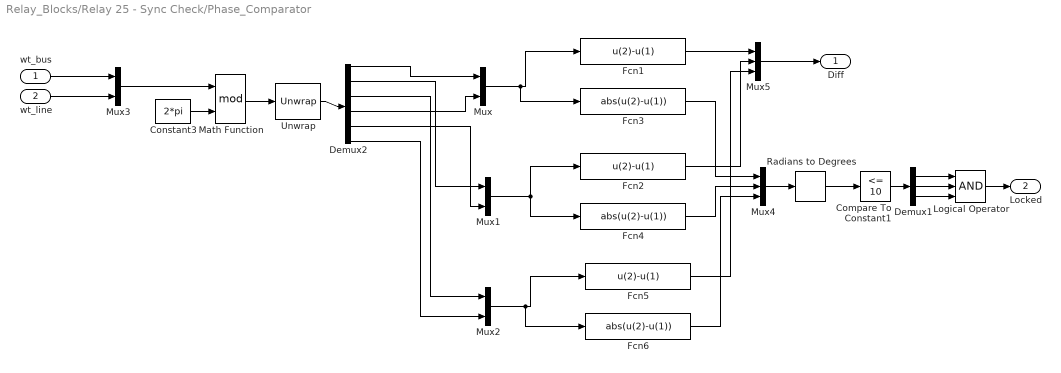
== system Relay_Blocks/Relay 25 - Sync Check/Phase_Comparator ==
  wt_bus : Inport
  wt_line : Inport  Port=2
  Compare To Constant1 : simulink/Logic and Bit Operations/Compare To Constant  relop=<=  const=10  OutDataTypeStr=uint8
  Constant3 : Constant  Value=2*pi
  Demux1 : Demux  Outputs=3
  Demux2 : Demux  Outputs=6
  Fcn1 : Fcn  Expr=u(2)-u(1)  SampleTime=Ts
  Fcn2 : Fcn  Expr=u(2)-u(1)  SampleTime=Ts
  Fcn3 : Fcn  Expr=abs(u(2)-u(1))  SampleTime=Ts
  Fcn4 : Fcn  Expr=abs(u(2)-u(1))  SampleTime=Ts
  Fcn5 : Fcn  Expr=u(2)-u(1)  SampleTime=Ts
  Fcn6 : Fcn  Expr=abs(u(2)-u(1))  SampleTime=Ts
  Logical Operator : Logic  Inputs=3  AllPortsSameDT=off  OutDataTypeStr=boolean
  Math Function : Math  Operator=mod  SampleTime=Ts  SaturateOnIntegerOverflow=on
  Mux{,1..3} (4 alike) : Mux  Inputs=2
  Mux4 : Mux  Inputs=3
  Mux5 : Mux  Inputs=3
  Radians to Degrees : simulink_extras/Transformations/Radians to Degrees
  Unwrap : dspsigops/Unwrap  tol=pi  InputProcessing=Columns as channels (frame based)  running=off
  Diff : Outport
  Locked : Outport  Port=2
  wires:
  Math Function/1 -> Unwrap/1
  wt_line/1 -> Mux3/2
  wt_bus/1 -> Mux3/1
  Mux3/1 -> Math Function/1
  Constant3/1 -> Math Function/2
  Radians to Degrees/1 -> Compare To Constant1/1
  Unwrap/1 -> Demux2/1
  Demux2/2 -> Mux1/1
  Demux2/3 -> Mux2/1
  Demux2/4 -> Mux/2
  Demux2/5 -> Mux1/2
  Demux2/6 -> Mux2/2
  Mux/1 -> Fcn1/1, Fcn3/1
  Mux1/1 -> Fcn2/1, Fcn4/1
  Mux2/1 -> Fcn5/1, Fcn6/1
  Fcn3/1 -> Mux4/1
  Fcn4/1 -> Mux4/2
  Fcn6/1 -> Mux4/3
  Mux4/1 -> Radians to Degrees/1
  Fcn1/1 -> Mux5/1
  Fcn2/1 -> Mux5/2
  Fcn5/1 -> Mux5/3
  Mux5/1 -> Diff/1
  Demux1/2 -> Logical Operator/2
  Demux1/3 -> Logical Operator/3
  Compare To Constant1/1 -> Demux1/1
  Demux1/1 -> Logical Operator/1
  Logical Operator/1 -> Locked/1
  Demux2/1 -> Mux/1

== system Relay_Blocks/Relay 25 - Sync Check/RMS Calculator1 ==
  Vpeak : Inport
  Constant9 : Constant  Value=sqrt(3)
  Discrete  Mean value6 : powerlib_extras/Discrete Measurements/Discrete  Mean value  Freq=60  Vinit=0  Ts=Ts
  Product1 : Product  SampleTime=Ts  RndMeth=Zero
  Product3 : Product  SampleTime=Ts  RndMeth=Zero
  Signed Sqrt : Sqrt  SampleTime=Ts  SaturateOnIntegerOverflow=on
  VRMSLL : Outport
  wires:
  Signed Sqrt/1 -> VRMSLL/1
  Vpeak/1 -> Product1/1
  Product1/1 -> Product3/1, Product3/2
  Constant9/1 -> Product1/2
  Product3/1 -> Discrete  Mean value6/1
  Discrete  Mean value6/1 -> Signed Sqrt/1

== system Relay_Blocks/Relay 25 - Sync Check/RMS Calculator2 ==
  Vpeak : Inport
  Constant9 : Constant  Value=sqrt(3)
  Discrete  Mean value6 : powerlib_extras/Discrete Measurements/Discrete  Mean value  Freq=60  Vinit=0  Ts=Ts
  Product1 : Product  SampleTime=Ts  RndMeth=Zero
  Product3 : Product  SampleTime=Ts  RndMeth=Zero
  Signed Sqrt : Sqrt  SampleTime=Ts  SaturateOnIntegerOverflow=on
  VRMSLL : Outport
  wires:
  Signed Sqrt/1 -> VRMSLL/1
  Vpeak/1 -> Product1/1
  Product1/1 -> Product3/1, Product3/2
  Constant9/1 -> Product1/2
  Product3/1 -> Discrete  Mean value6/1
  Discrete  Mean value6/1 -> Signed Sqrt/1

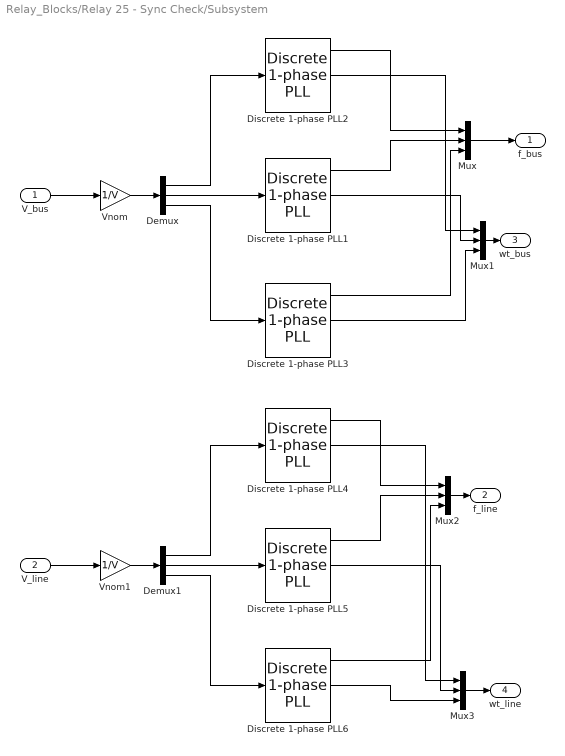
== system Relay_Blocks/Relay 25 - Sync Check/Subsystem ==
  V_bus : Inport
  V_line : Inport  Port=2
  Demux : Demux  Outputs=3
  Demux1 : Demux  Outputs=3
  Discrete 1-phase PLL{1..6} (6 alike) : powerlib_extras/Discrete  Control Blocks/Discrete 1-phase PLL  Fmin=45  Par_Init=[0 60]  ParK=[ 180 3200 1]  Ts=50e-6  AGC=on
  Mux{,1..3} (4 alike) : Mux  Inputs=3
  Vnom : Gain  Gain=1/V
  Vnom1 : Gain  Gain=1/V
  f_bus : Outport
  f_line : Outport  Port=2
  wt_bus : Outport  Port=3
  wt_line : Outport  Port=4
  wires:
  V_line/1 -> Vnom1/1
  Vnom/1 -> Demux/1
  Vnom1/1 -> Demux1/1
  Demux1/1 -> Discrete 1-phase PLL4/1
  Demux1/2 -> Discrete 1-phase PLL5/1
  Demux1/3 -> Discrete 1-phase PLL6/1
  Demux/1 -> Discrete 1-phase PLL2/1
  Demux/2 -> Discrete 1-phase PLL1/1
  Demux/3 -> Discrete 1-phase PLL3/1
  Discrete 1-phase PLL2/1 -> Mux/1
  Discrete 1-phase PLL1/1 -> Mux/2
  Discrete 1-phase PLL3/1 -> Mux/3
  Mux/1 -> f_bus/1
  Discrete 1-phase PLL2/2 -> Mux1/1
  Discrete 1-phase PLL1/2 -> Mux1/2
  Discrete 1-phase PLL3/2 -> Mux1/3
  Mux1/1 -> wt_bus/1
  Discrete 1-phase PLL4/1 -> Mux2/1
  Discrete 1-phase PLL6/1 -> Mux2/3
  Discrete 1-phase PLL5/1 -> Mux2/2
  Discrete 1-phase PLL4/2 -> Mux3/1
  Discrete 1-phase PLL5/2 -> Mux3/2
  Discrete 1-phase PLL6/2 -> Mux3/3
  Mux2/1 -> f_line/1
  Mux3/1 -> wt_line/1
  V_bus/1 -> Vnom/1

== system Relay_Blocks/Relay 25 - Sync Check/Voltage_Comparator ==
  V_bus : Inport
  V_line : Inport  Port=2
  Compare To Constant : simulink/Logic and Bit Operations/Compare To Constant  relop=<=  const=414  OutDataTypeStr=uint8
  Discrete Transfer Fcn : DiscreteTransferFcn  Numerator=[0.0004999]  Denominator=[1 -0.9995]  SampleTime=-1
  Fcn2 : Fcn  Expr=abs(u(2)-u(1))
  Mux1 : Mux  Inputs=2
  Diff : Outport
  Filt_Diff : Outport  Port=2
  Locked : Outport  Port=3
  wires:
  V_bus/1 -> Mux1/1
  V_line/1 -> Mux1/2
  Discrete Transfer Fcn/1 -> Compare To Constant/1, Filt_Diff/1
  Compare To Constant/1 -> Locked/1
  Fcn2/1 -> Diff/1, Discrete Transfer Fcn/1
  Mux1/1 -> Fcn2/1

== system Relay_Blocks/Relay 27 - UV/UV Relay ==
  TOV_pickup : Inport
  Va : Inport  Port=2
  Vb : Inport  Port=3
  Vc : Inport  Port=4
  Demux1 : Demux  Outputs=3
  Divide : Product  Inputs=*/
  IEC Std : Fcn  Expr=(0.14/ (1 - u(1)^0.050 ))
  IEC Std1 : Fcn  Expr=(0.14/ (1 - u(1)^0.050 ))
  IEC Std2 : Fcn  Expr=(0.14/ (1 - u(1)^0.050 ))
  MinMax : MinMax
  Mux : Mux  Inputs=3
  Mux1 : Mux  Inputs=3
  f : Fcn  Expr=(u(1)>0)*u(1)/(u(1)>0)
  f1 : Fcn  Expr=(u(1)>0)*u(1)/(u(1)>0)
  f2 : Fcn  Expr=(u(1)>0)*u(1)/(u(1)>0)
  T_trip : Outport
  wires:
  Vc/1 -> Mux/3
  TOV_pickup/1 -> Divide/2
  MinMax/1 -> T_trip/1
  Vb/1 -> Mux/2
  Va/1 -> Mux/1
  f2/1 -> Mux1/3
  f1/1 -> Mux1/2
  f/1 -> Mux1/1
  Mux/1 -> Divide/1
  Mux1/1 -> MinMax/1
  IEC Std2/1 -> f2/1
  IEC Std1/1 -> f1/1
  IEC Std/1 -> f/1
  Divide/1 -> Demux1/1
  Demux1/3 -> IEC Std2/1
  Demux1/2 -> IEC Std1/1
  Demux1/1 -> IEC Std/1

== system Relay_Blocks/Relay 59 - OV/OV Relay ==
  TOV_pickup : Inport
  Va : Inport  Port=2
  Vb : Inport  Port=3
  Vc : Inport  Port=4
  Demux1 : Demux  Outputs=3
  Divide : Product  Inputs=*/
  IEC Std : Fcn  Expr=(0.14/ (u(1)^0.050 - 1))
  IEC Std1 : Fcn  Expr=(0.14/ (u(1)^0.050 - 1))
  IEC Std2 : Fcn  Expr=(0.14/ (u(1)^0.050 - 1))
  MinMax : MinMax
  Mux : Mux  Inputs=3
  Mux1 : Mux  Inputs=3
  f : Fcn  Expr=(u(1)>0)*u(1)/(u(1)>0)
  f1 : Fcn  Expr=(u(1)>0)*u(1)/(u(1)>0)
  f2 : Fcn  Expr=(u(1)>0)*u(1)/(u(1)>0)
  T_trip : Outport
  wires:
  Vc/1 -> Mux/3
  TOV_pickup/1 -> Divide/2
  MinMax/1 -> T_trip/1
  Vb/1 -> Mux/2
  Va/1 -> Mux/1
  Mux/1 -> Divide/1
  Mux1/1 -> MinMax/1
  IEC Std2/1 -> f2/1
  IEC Std1/1 -> f1/1
  IEC Std/1 -> f/1
  Divide/1 -> Demux1/1
  Demux1/3 -> IEC Std2/1
  Demux1/2 -> IEC Std1/1
  Demux1/1 -> IEC Std/1
  f2/1 -> Mux1/3
  f1/1 -> Mux1/2
  f/1 -> Mux1/1

== system Relay_Blocks/Old_13.8kV Gen - IEEE 1547/Frequency1/If Action Subsystem11 ==
  In1 : Inport
  Action Port : ActionPort  ActionType=else
  Out1 : Outport
  wires:
  In1/1 -> Out1/1

== system Relay_Blocks/Old_13.8kV Gen - IEEE 1547/Frequency1/If Action Subsystem6 ==
  In1 : Inport
  Action Port : ActionPort  ActionType=then
  Out1 : Outport
  wires:
  In1/1 -> Out1/1

== system Relay_Blocks/Old_13.8kV Gen - IEEE 1547/Frequency1/If Action Subsystem7 ==
  In1 : Inport
  Action Port : ActionPort  ActionType=elseif
  Out1 : Outport
  wires:
  In1/1 -> Out1/1

== system Relay_Blocks/Old_13.8kV Gen - IEEE 1547/Frequency1/If Action Subsystem8 ==
  In1 : Inport
  Action Port : ActionPort  ActionType=elseif
  Out1 : Outport
  wires:
  In1/1 -> Out1/1

== system Relay_Blocks/Old_13.8kV Gen - IEEE 1547/Frequency1/If Action Subsystem9 ==
  In1 : Inport
  Action Port : ActionPort  ActionType=elseif
  Out1 : Outport
  wires:
  In1/1 -> Out1/1

== system Relay_Blocks/Old_13.8kV Gen - IEEE 1547/PhaseA/If Action Subsystem ==
  In1 : Inport
  Action Port : ActionPort  ActionType=then
  Out1 : Outport
  wires:
  In1/1 -> Out1/1

== system Relay_Blocks/Old_13.8kV Gen - IEEE 1547/PhaseA/If Action Subsystem1 ==
  In1 : Inport
  Action Port : ActionPort  ActionType=elseif
  Out1 : Outport
  wires:
  In1/1 -> Out1/1

== system Relay_Blocks/Old_13.8kV Gen - IEEE 1547/PhaseA/If Action Subsystem2 ==
  In1 : Inport
  Action Port : ActionPort  ActionType=elseif
  Out1 : Outport
  wires:
  In1/1 -> Out1/1

== system Relay_Blocks/Old_13.8kV Gen - IEEE 1547/PhaseA/If Action Subsystem3 ==
  In1 : Inport
  Action Port : ActionPort  ActionType=elseif
  Out1 : Outport
  wires:
  In1/1 -> Out1/1

== system Relay_Blocks/Old_13.8kV Gen - IEEE 1547/PhaseA/If Action Subsystem4 ==
  In1 : Inport
  Action Port : ActionPort  ActionType=elseif
  Out1 : Outport
  wires:
  In1/1 -> Out1/1

== system Relay_Blocks/Old_13.8kV Gen - IEEE 1547/PhaseA/If Action Subsystem5 ==
  In1 : Inport
  Action Port : ActionPort  ActionType=else
  Out1 : Outport
  wires:
  In1/1 -> Out1/1

== system Relay_Blocks/Old_13.8kV Gen - IEEE 1547/PhaseB/If Action Subsystem ==
  In1 : Inport
  Action Port : ActionPort  ActionType=then
  Out1 : Outport
  wires:
  In1/1 -> Out1/1

== system Relay_Blocks/Old_13.8kV Gen - IEEE 1547/PhaseB/If Action Subsystem1 ==
  In1 : Inport
  Action Port : ActionPort  ActionType=elseif
  Out1 : Outport
  wires:
  In1/1 -> Out1/1

== system Relay_Blocks/Old_13.8kV Gen - IEEE 1547/PhaseB/If Action Subsystem2 ==
  In1 : Inport
  Action Port : ActionPort  ActionType=elseif
  Out1 : Outport
  wires:
  In1/1 -> Out1/1

== system Relay_Blocks/Old_13.8kV Gen - IEEE 1547/PhaseB/If Action Subsystem3 ==
  In1 : Inport
  Action Port : ActionPort  ActionType=elseif
  Out1 : Outport
  wires:
  In1/1 -> Out1/1

== system Relay_Blocks/Old_13.8kV Gen - IEEE 1547/PhaseB/If Action Subsystem4 ==
  In1 : Inport
  Action Port : ActionPort  ActionType=elseif
  Out1 : Outport
  wires:
  In1/1 -> Out1/1

== system Relay_Blocks/Old_13.8kV Gen - IEEE 1547/PhaseB/If Action Subsystem5 ==
  In1 : Inport
  Action Port : ActionPort  ActionType=else
  Out1 : Outport
  wires:
  In1/1 -> Out1/1

== system Relay_Blocks/Old_13.8kV Gen - IEEE 1547/PhaseC/If Action Subsystem ==
  In1 : Inport
  Action Port : ActionPort  ActionType=then
  Out1 : Outport
  wires:
  In1/1 -> Out1/1

== system Relay_Blocks/Old_13.8kV Gen - IEEE 1547/PhaseC/If Action Subsystem1 ==
  In1 : Inport
  Action Port : ActionPort  ActionType=elseif
  Out1 : Outport
  wires:
  In1/1 -> Out1/1

== system Relay_Blocks/Old_13.8kV Gen - IEEE 1547/PhaseC/If Action Subsystem2 ==
  In1 : Inport
  Action Port : ActionPort  ActionType=elseif
  Out1 : Outport
  wires:
  In1/1 -> Out1/1

== system Relay_Blocks/Old_13.8kV Gen - IEEE 1547/PhaseC/If Action Subsystem3 ==
  In1 : Inport
  Action Port : ActionPort  ActionType=elseif
  Out1 : Outport
  wires:
  In1/1 -> Out1/1

== system Relay_Blocks/Old_13.8kV Gen - IEEE 1547/PhaseC/If Action Subsystem4 ==
  In1 : Inport
  Action Port : ActionPort  ActionType=elseif
  Out1 : Outport
  wires:
  In1/1 -> Out1/1

== system Relay_Blocks/Old_13.8kV Gen - IEEE 1547/PhaseC/If Action Subsystem5 ==
  In1 : Inport
  Action Port : ActionPort  ActionType=else
  Out1 : Outport
  wires:
  In1/1 -> Out1/1

== system Relay_Blocks/Old_460V Gen - IEEE 1547/Frequency1/If Action Subsystem11 ==
  In1 : Inport
  Action Port : ActionPort  ActionType=else
  Out1 : Outport
  wires:
  In1/1 -> Out1/1

== system Relay_Blocks/Old_460V Gen - IEEE 1547/Frequency1/If Action Subsystem6 ==
  In1 : Inport
  Action Port : ActionPort  ActionType=then
  Out1 : Outport
  wires:
  In1/1 -> Out1/1

== system Relay_Blocks/Old_460V Gen - IEEE 1547/Frequency1/If Action Subsystem7 ==
  In1 : Inport
  Action Port : ActionPort  ActionType=elseif
  Out1 : Outport
  wires:
  In1/1 -> Out1/1

== system Relay_Blocks/Old_460V Gen - IEEE 1547/Frequency1/If Action Subsystem8 ==
  In1 : Inport
  Action Port : ActionPort  ActionType=elseif
  Out1 : Outport
  wires:
  In1/1 -> Out1/1

== system Relay_Blocks/Old_460V Gen - IEEE 1547/Frequency1/If Action Subsystem9 ==
  In1 : Inport
  Action Port : ActionPort  ActionType=elseif
  Out1 : Outport
  wires:
  In1/1 -> Out1/1

== system Relay_Blocks/Old_460V Gen - IEEE 1547/PhaseA/If Action Subsystem ==
  In1 : Inport
  Action Port : ActionPort  ActionType=then
  Out1 : Outport
  wires:
  In1/1 -> Out1/1

== system Relay_Blocks/Old_460V Gen - IEEE 1547/PhaseA/If Action Subsystem1 ==
  In1 : Inport
  Action Port : ActionPort  ActionType=elseif
  Out1 : Outport
  wires:
  In1/1 -> Out1/1

== system Relay_Blocks/Old_460V Gen - IEEE 1547/PhaseA/If Action Subsystem2 ==
  In1 : Inport
  Action Port : ActionPort  ActionType=elseif
  Out1 : Outport
  wires:
  In1/1 -> Out1/1

== system Relay_Blocks/Old_460V Gen - IEEE 1547/PhaseA/If Action Subsystem3 ==
  In1 : Inport
  Action Port : ActionPort  ActionType=elseif
  Out1 : Outport
  wires:
  In1/1 -> Out1/1

== system Relay_Blocks/Old_460V Gen - IEEE 1547/PhaseA/If Action Subsystem4 ==
  In1 : Inport
  Action Port : ActionPort  ActionType=elseif
  Out1 : Outport
  wires:
  In1/1 -> Out1/1

== system Relay_Blocks/Old_460V Gen - IEEE 1547/PhaseA/If Action Subsystem5 ==
  In1 : Inport
  Action Port : ActionPort  ActionType=else
  Out1 : Outport
  wires:
  In1/1 -> Out1/1

== system Relay_Blocks/Old_460V Gen - IEEE 1547/PhaseB/If Action Subsystem ==
  In1 : Inport
  Action Port : ActionPort  ActionType=then
  Out1 : Outport
  wires:
  In1/1 -> Out1/1

== system Relay_Blocks/Old_460V Gen - IEEE 1547/PhaseB/If Action Subsystem1 ==
  In1 : Inport
  Action Port : ActionPort  ActionType=elseif
  Out1 : Outport
  wires:
  In1/1 -> Out1/1

== system Relay_Blocks/Old_460V Gen - IEEE 1547/PhaseB/If Action Subsystem2 ==
  In1 : Inport
  Action Port : ActionPort  ActionType=elseif
  Out1 : Outport
  wires:
  In1/1 -> Out1/1

== system Relay_Blocks/Old_460V Gen - IEEE 1547/PhaseB/If Action Subsystem3 ==
  In1 : Inport
  Action Port : ActionPort  ActionType=elseif
  Out1 : Outport
  wires:
  In1/1 -> Out1/1

== system Relay_Blocks/Old_460V Gen - IEEE 1547/PhaseB/If Action Subsystem4 ==
  In1 : Inport
  Action Port : ActionPort  ActionType=elseif
  Out1 : Outport
  wires:
  In1/1 -> Out1/1

== system Relay_Blocks/Old_460V Gen - IEEE 1547/PhaseB/If Action Subsystem5 ==
  In1 : Inport
  Action Port : ActionPort  ActionType=else
  Out1 : Outport
  wires:
  In1/1 -> Out1/1

== system Relay_Blocks/Old_460V Gen - IEEE 1547/PhaseC/If Action Subsystem ==
  In1 : Inport
  Action Port : ActionPort  ActionType=then
  Out1 : Outport
  wires:
  In1/1 -> Out1/1

== system Relay_Blocks/Old_460V Gen - IEEE 1547/PhaseC/If Action Subsystem1 ==
  In1 : Inport
  Action Port : ActionPort  ActionType=elseif
  Out1 : Outport
  wires:
  In1/1 -> Out1/1

== system Relay_Blocks/Old_460V Gen - IEEE 1547/PhaseC/If Action Subsystem2 ==
  In1 : Inport
  Action Port : ActionPort  ActionType=elseif
  Out1 : Outport
  wires:
  In1/1 -> Out1/1

== system Relay_Blocks/Old_460V Gen - IEEE 1547/PhaseC/If Action Subsystem3 ==
  In1 : Inport
  Action Port : ActionPort  ActionType=elseif
  Out1 : Outport
  wires:
  In1/1 -> Out1/1

== system Relay_Blocks/Old_460V Gen - IEEE 1547/PhaseC/If Action Subsystem4 ==
  In1 : Inport
  Action Port : ActionPort  ActionType=elseif
  Out1 : Outport
  wires:
  In1/1 -> Out1/1

== system Relay_Blocks/Old_460V Gen - IEEE 1547/PhaseC/If Action Subsystem5 ==
  In1 : Inport
  Action Port : ActionPort  ActionType=else
  Out1 : Outport
  wires:
  In1/1 -> Out1/1

== matlab function IEEE 1547 V&F/Over/Under Voltage/Frequency ==
  data: resetVoltage output double; Voltage_Trip_time output double; resetFreq output double; v input double; Frequency_Trip_time output double; va input double; vb input double; vc input double; freq input double; OF1 input double; OF2 input double; UF1 input double; UF2 input double; OV1 input double; OV2 input double; UV1 input double; UV2 input double; UV3 input double
function [  resetVoltage, Voltage_Trip_time, resetFreq, Frequency_Trip_time] = fcn(v, va, vb, vc, freq, OF1, OF2, UF1, UF2, OV1, OV2, UV1, UV2, UV3)

%This function implements time over/under voltage and over/under frequency.
%The clearing times are able to be set via the mask of the block.


resetA = 0;
resetB = 0;
resetC = 0;
resetFreq = 0;
timeA = inf;
timeB = inf;
timeC = inf;

if(0.45*v > va)
    timeA = UV1;
elseif((0.45*v <= va) && (va < 0.6*v))
    timeA = UV2;
elseif((0.6*v <= va) && (va < 0.88*v))
    timeA = UV3;
elseif((1.1*v < va) && (va < 1.2*v))
    timeA = OV1;
elseif(1.2*v < va)
    timeA = OV2;
else
    timeA = inf;
    resetA = 1;
end

if(0.45*v > vb)
    timeB = UV1;
elseif((0.45*v <= vb) && (vb < 0.6*v))
    timeB = UV2;
elseif((0.6*v <= vb) && (vb < 0.88*v))
    timeB = UV3;
elseif((1.1*v < vb) && (vb < 1.2*v))
    timeB = OV1;
elseif(1.2*v < vb)
    timeB = OV2;
else
    timeB = inf;
    resetB = 1;
end

if(0.45*v > vc)
    timeC = UV1;
elseif((0.45*v <= vc) && (vc < 0.6*v))
    timeC = UV2;
elseif((0.6*v <= vc) && (vc < 0.88*v))
    timeC = UV3;
elseif((1.1*v < vc) && (vc < 1.2*v))
    timeC = OV1;
elseif(1.2*v < vc)
    timeC = OV2;
else
    timeC = inf;
    resetC = 1;
end

if(freq <57)
    timeFreq = UF1;
elseif((57 <= freq) && (freq < 59.5))
    timeFreq = UF2;
elseif((60.5 <= freq) && (freq < 62))
    timeFreq = OF1;
elseif(freq >= 62)
    timeFreq = OF2;
else
    timeFreq = inf;
    resetFreq = 1;
end

time_vector = [timeA timeB timeC];
Voltage_Trip_time = min(time_vector);
Frequency_Trip_time = timeFreq;
resetVoltage = resetA & resetB & resetC;  %want to always reset timer time when all voltages are acceptable
